simulink model "PassengerCar"  (R2019b)
settings: Solver=ode1  StartTime=0  StopTime=25  FixedStep=1.0000000000000000e-003  RelTol=1e-3
InitFcn:
  | sampleTime = str2double(get_param(bdroot, 'FixedStep'));
undefined symbols (not defined in the file or in its folder): AccPedalPos, BrakePedalPos, BrakeSwitch, DiscIntNeverNeededParam, DYNA4, EngSpd, IgnitionSwitch, InitialGear, InitialSpeed, IntendedEngTrq, LeftIndicator, MainBrakePress, MaxGear, MDL, MinGear, RefAcc, RefLane, RefLatPos, RefPath, RefPathCurv, RefSpd, RefSpdPreview, RefSpdRetrospect, RightIndicator, SteeringWheelAng, SteeringWheelTrq, UserDefinedRefValue, vm_const
libraries: UtilitiesLibrary x31, simulink x18, WheelSystemModules x13, LongitudinalControllerModules x13, LateralControllerModules x7, AnimationBusselectorModules x5, EnvironmentModules x5, BasicEngineControlModules x5, MiscellaneousControlModules x5, Animation3Modules x4, AuxiliariesModules x4, TireModules x4
(part 17 of 39)

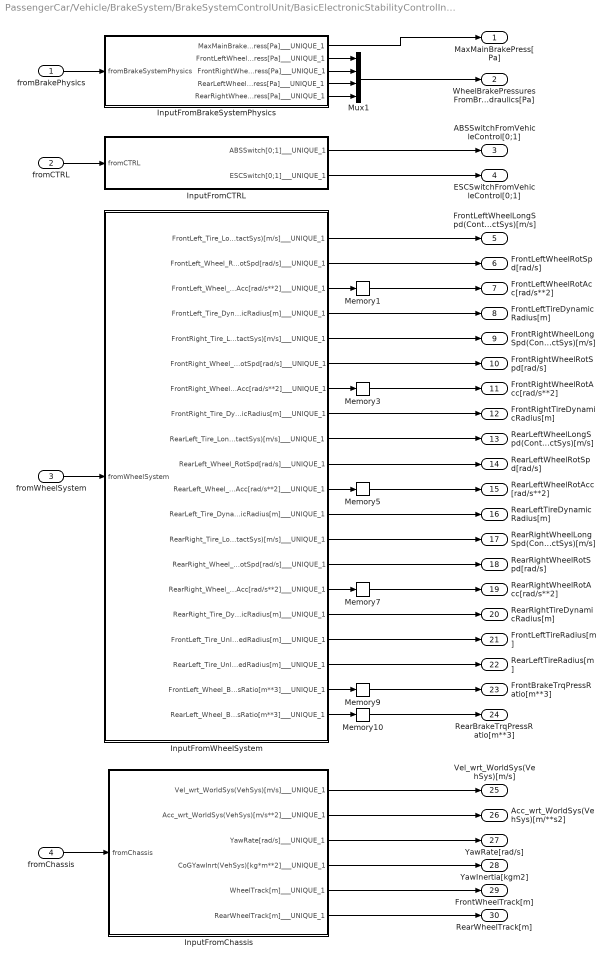
== system PassengerCar/Vehicle/BrakeSystem/BrakeSystemControlUnit/BasicElectronicStabilityControlInput ==
  fromBrakePhysics : Inport
  fromCTRL : Inport  Port=2
  fromWheelSystem : Inport  Port=3
  fromChassis : Inport  Port=4
  InputFromBrakeSystemPhysics : Subsystem  Tag=TESIS DYNAware Interface Block  mask{NeedsUpdate=off, SignalInfo=|}
      mask SignalInfo=|
      | {
      |   "Version": "4.6",
      |   "MuxedOutputBusName": "output",
      |   "MuxedInputBusName": "fromBrakeSystemPhysics",
      |   "MuxedInputSelected": true,
      |   "MuxedOutputSelected": false,
      |   "SignalData": [
      |     {
      |       "initialValue": "",
      |       "name": "MaxMainBrakePress[Pa]",
      |       "comment": "",
      |       "minString": "",
      |       "maxString": "",
      |       "width": -1,
      |       "dataType": 0,
      |       "signalType": 0,
      |       "createSignal": false,
      |       "outputName": "MaxMainBrakePress[Pa]",
      |       "generateSignalAccessBlock": false,
      |       "accessId": "$(parentId).$(blockName).$(outputName)"
      |     },
      |     {
      |       "initialValue": "",
      |       "name": "FrontLeftWheelBrakePress[Pa]",
      |       "comment": "",
      |       "minString": "",
      |       "maxString": "",
      |       "width": -1,
      |       "dataType": 0,
      |       "signalType": 0,
      |       "createSignal": false,
      |       "outputName": "FrontLeftWheelBrakePress[Pa]",
      |       "generateSignalAccessBlock": false,
      |       "accessId": "$(parentId).$(blockName).$(outputName)"
      |     },
      |     {
      |       "initialValue": "",
      |       "name": "FrontRightWheelBrakePress[Pa]",
      |       "comment": "",
      |       "minString": "",
      |       "maxString": "",
      |       "width": -1,
      |       "dataType": 0,
      |       "signalType": 0,
      |       "createSignal": false,
      |       "outputName": "FrontRightWheelBrakePress[Pa]",
      |       "generateSignalAccessBlock": false,
      |       "accessId": "$(parentId).$(blockName).$(outputName)"
      |     },
      |     {
      |       "initialValue": "",
      |       "name": "RearLeftWheelBrakePress[Pa]",
      |       "comment": "",
      |       "minString": "",
      |       "maxString": "",
      |       "width": -1,
      |       "dataType": 0,
      |       "signalType": 0,
      |       "createSignal": false,
      |       "outputName": "RearLeftWheelBrakePress[Pa]",
      |       "generateSignalAccessBlock": false,
      |       "accessId": "$(parentId).$(blockName).$(outputName)"
      |     },
      |     {
      |       "initialValue": "",
      |       "name": "RearRightWheelBrakePress[Pa]",
      |       "comment": "",
      |       "minString": "",
      |       "maxString": "",
      |       "width": -1,
      |       "dataType": 0,
      |       "signalType": 0,
      |       "createSignal": false,
      |       "outputName": "RearRightWheelBrakePress[Pa]",
      |       "generateSignalAccessBlock": false,
      |       "accessId": "$(parentId).$(blockName).$(outputName)"
      |     }
      |   ]
      | }
      mask prompts: NeedsUpdate "Specify, if subsystem content needs to be updated"; SignalInfo "Signal Info (json)"
      mask help: DYNA4 Interface Block Version 4.6
      mask init:
      | blockName = get_param(gcbh, 'Name');
      | parentId = DYNA4.ModelHandling.AccessID.getFromHierarchy(gcbh);
      | TD.InterfaceBlock.ModelCallbacks.GenerateContent(gcb);
      settings: DeleteFcn=TD.InterfaceBlock.ModelCallbacks.CloseGUI( gcbh );  NameChangeFcn=TD.InterfaceBlock.ModelCallbacks.BlockRenamedHandler(gcbh);  OpenFcn=TD.InterfaceBlock.ModelCallbacks.OpenGUI( gcbh );  CloseFcn=TD.InterfaceBlock.ModelCallbacks.CloseGUI( gcbh );
      mask Display:
      | image('InterfaceBlock.png','center');
      | port_label('input',1, 'fromBrakeSystemPhysics');
      | port_label('output',1, 'MaxMainBrakePress[Pa]');
      | port_label('output',2, 'FrontLeftWheelBrakePress[Pa]');
      | port_label('output',3, 'FrontRightWheelBrakePress[Pa]');
      | port_label('output',4, 'RearLeftWheelBrakePress[Pa]');
      | port_label('output',5, 'RearRightWheelBrakePress[Pa]');
  InputFromCTRL : Subsystem  Tag=TESIS DYNAware Interface Block  mask{NeedsUpdate=off, SignalInfo=|}
      mask SignalInfo=|
      | {
      |   "Version": "4.6",
      |   "MuxedOutputBusName": "output",
      |   "MuxedInputBusName": "fromCTRL",
      |   "MuxedInputSelected": true,
      |   "MuxedOutputSelected": false,
      |   "SignalData": [
      |     {
      |       "initialValue": "0.0",
      |       "name": "CTRL.LongitudinalControl.ABSSwitch[0;1]",
      |       "comment": "",
      |       "minString": "",
      |       "maxString": "",
      |       "width": 1,
      |       "dataType": 0,
      |       "signalType": 0,
      |       "createSignal": false,
      |       "outputName": "ABSSwitch[0;1]",
      |       "generateSignalAccessBlock": false,
      |       "accessId": "$(parentId).$(blockName).$(outputName)"
      |     },
      |     {
      |       "initialValue": "0.0",
      |       "name": "CTRL.LongitudinalControl.ESCSwitch[0;1]",
      |       "comment": "",
      |       "minString": "",
      |       "maxString": "",
      |       "width": 1,
      |       "dataType": 0,
      |       "signalType": 0,
      |       "createSignal": false,
      |       "outputName": "ESCSwitch[0;1]",
      |       "generateSignalAccessBlock": false,
      |       "accessId": "$(parentId).$(blockName).$(outputName)"
      |     }
      |   ]
      | }
      mask prompts: NeedsUpdate "Specify, if subsystem content needs to be updated"; SignalInfo "Signal Info (json)"
      mask help: DYNA4 Interface Block Version 4.6
      mask init:
      | blockName = get_param(gcbh, 'Name');
      | parentId = DYNA4.ModelHandling.AccessID.getFromHierarchy(gcbh);
      | TD.InterfaceBlock.ModelCallbacks.GenerateContent(gcb);
      settings: DeleteFcn=TD.InterfaceBlock.ModelCallbacks.CloseGUI( gcbh );  NameChangeFcn=TD.InterfaceBlock.ModelCallbacks.BlockRenamedHandler(gcbh);  OpenFcn=TD.InterfaceBlock.ModelCallbacks.OpenGUI( gcbh );  CloseFcn=TD.InterfaceBlock.ModelCallbacks.CloseGUI( gcbh );
      mask Display:
      | image('InterfaceBlock.png','center');
      | port_label('input',1, 'fromCTRL');
      | port_label('output',1, 'ABSSwitch[0;1]');
      | port_label('output',2, 'ESCSwitch[0;1]');
  InputFromChassis : Subsystem  Tag=TESIS DYNAware Interface Block  mask{NeedsUpdate=off, SignalInfo=|}
      mask SignalInfo=|
      | {
      |   "Version": "4.6",
      |   "MuxedOutputBusName": "output",
      |   "MuxedInputBusName": "fromChassis",
      |   "MuxedInputSelected": true,
      |   "MuxedOutputSelected": false,
      |   "SignalData": [
      |     {
      |       "initialValue": "0.0",
      |       "name": "VehicleBody.Vel_wrt_WorldSys(VehSys)[m/s]",
      |       "comment": "",
      |       "minString": "",
      |       "maxString": "",
      |       "width": 3,
      |       "dataType": 0,
      |       "signalType": 0,
      |       "createSignal": false,
      |       "outputName": "Vel_wrt_WorldSys(VehSys)[m/s]",
      |       "generateSignalAccessBlock": false,
      |       "accessId": "$(parentId).$(blockName).$(outputName)"
      |     },
      |     {
      |       "initialValue": "0.0",
      |       "name": "VehicleBody.Acc_wrt_WorldSys(VehSys)[m/s**2]",
      |       "comment": "",
      |       "minString": "",
      |       "maxString": "",
      |       "width": 3,
      |       "dataType": 0,
      |       "signalType": 0,
      |       "createSignal": false,
      |       "outputName": "Acc_wrt_WorldSys(VehSys)[m/s**2]",
      |       "generateSignalAccessBlock": false,
      |       "accessId": "$(parentId).$(blockName).$(outputName)"
      |     },
      |     {
      |       "initialValue": "0.0",
      |       "name": "VehicleBody.YawRate[rad/s]",
      |       "comment": "",
      |       "minString": "",
      |       "maxString": "",
      |       "width": 1,
      |       "dataType": 0,
      |       "signalType": 0,
      |       "createSignal": false,
      |       "outputName": "YawRate[rad/s]",
      |       "generateSignalAccessBlock": false,
      |       "accessId": "$(parentId).$(blockName).$(outputName)"
      |     },
      |     {
      |       "initialValue": "0.0",
      |       "name": "VehicleBody.CoGYawInrt(VehSys)[kg*m**2]",
      |       "comment": "",
      |       "minString": "",
      |       "maxString": "",
      |       "width": 1,
      |       "dataType": 0,
      |       "signalType": 0,
      |       "createSignal": false,
      |       "outputName": "CoGYawInrt(VehSys)[kg*m**2]",
      |       "generateSignalAccessBlock": false,
      |       "accessId": "$(parentId).$(blockName).$(outputName)"
      |     },
      |     {
      |       "initialValue": "0.0",
      |       "name": "FrontAxle.WheelTrack[m]",
      |       "comment": "",
      |       "minString": "",
      |       "maxString": "",
      |       "width": 1,
      |       "dataType": 0,
      |       "signalType": 0,
      |       "createSignal": false,
      |       "outputName": "WheelTrack[m]",
      |       "generateSignalAccessBlock": false,
      |       "accessId": "$(parentId).$(blockName).$(outputName)"
      |     },
      |     {
      |       "initialValue": "0.0",
      |       "name": "RearAxle.WheelTrack[m]",
      |       "comment": "",
      |       "minString": "",
      |       "maxString": "",
      |       "width": 1,
      |       "dataType": 0,
      |       "signalType": 0,
      |       "createSignal": false,
      |       "outputName": "RearWheelTrack[m]",
      |       "generateSignalAccessBlock": false,
      |       "accessId": "$(parentId).$(blockName).$(outputName)"
      |     }
      |   ]
      | }
      mask prompts: NeedsUpdate "Specify, if subsystem content needs to be updated"; SignalInfo "Signal Info (json)"
      mask help: DYNA4 Interface Block Version 4.6
      mask init:
      | blockName = get_param(gcbh, 'Name');
      | parentId = DYNA4.ModelHandling.AccessID.getFromHierarchy(gcbh);
      | TD.InterfaceBlock.ModelCallbacks.GenerateContent(gcb);
      settings: DeleteFcn=TD.InterfaceBlock.ModelCallbacks.CloseGUI( gcbh );  NameChangeFcn=TD.InterfaceBlock.ModelCallbacks.BlockRenamedHandler(gcbh);  OpenFcn=TD.InterfaceBlock.ModelCallbacks.OpenGUI( gcbh );  CloseFcn=TD.InterfaceBlock.ModelCallbacks.CloseGUI( gcbh );
      mask Display:
      | image('InterfaceBlock.png','center');
      | port_label('input',1, 'fromChassis');
      | port_label('output',1, 'Vel_wrt_WorldSys(VehSys)[m/s]');
      | port_label('output',2, 'Acc_wrt_WorldSys(VehSys)[m/s**2]');
      | port_label('output',3, 'YawRate[rad/s]');
      | port_label('output',4, 'CoGYawInrt(VehSys)[kg*m**2]');
      | port_label('output',5, 'WheelTrack[m]');
      | port_label('output',6, 'RearWheelTrack[m]');
  InputFromWheelSystem : Subsystem  Tag=TESIS DYNAware Interface Block  mask{NeedsUpdate=off, SignalInfo=|}
      mask SignalInfo=|
      | {
      |   "Version": "4.6",
      |   "MuxedOutputBusName": "output",
      |   "MuxedInputBusName": "fromWheelSystem",
      |   "MuxedInputSelected": true,
      |   "MuxedOutputSelected": false,
      |   "SignalData": [
      |     {
      |       "initialValue": "0.0",
      |       "name": "FrontLeft.Tire.LongSpd(ContactSys)[m/s]",
      |       "comment": "Front left longitudinal wheel speed in contact system",
      |       "minString": "",
      |       "maxString": "",
      |       "width": 1,
      |       "dataType": 0,
      |       "signalType": 0,
      |       "createSignal": false,
      |       "outputName": "FrontLeft_Tire_LongSpd(ContactSys)[m/s]",
      |       "generateSignalAccessBlock": false,
      |       "accessId": "$(parentId).$(blockName).$(outputName)"
      |     },
      |     {
      |       "initialValue": "0.0",
      |       "name": "FrontLeft.Wheel.RotSpd[rad/s]",
      |       "comment": "Front left wheel rotational speed",
      |       "minString": "",
      |       "maxString": "",
      |       "width": -1,
      |       "dataType": 0,
      |       "signalType": 0,
      |       "createSignal": false,
      |       "outputName": "FrontLeft_Wheel_RotSpd[rad/s]",
      |       "generateSignalAccessBlock": false,
      |       "accessId": "$(parentId).$(blockName).$(outputName)"
      |     },
      |     {
      |       "initialValue": "0.0",
      |       "name": "FrontLeft.Wheel.RotAcc[rad/s**2]",
      |       "comment": "Front left wheel rotational acceleration",
      |       "minString": "",
      |       "maxString": "",
      |       "width": 1,
      |       "dataType": 0,
      |       "signalType": 0,
      |       "createSignal": false,
      |       "outputName": "FrontLeft_Wheel_RotAcc[rad/s**2]",
      |       "generateSignalAccessBlock": false,
      |       "accessId": "$(parentId).$(blockName).$(outputName)"
      |     },
      |     {
      |       "initialValue": "0.0",
      |       "name": "FrontLeft.Tire.DynamicRadius[m]",
      |       "comment": "Front left tire dynamic radius",
      |       "minString": "",
      |       "maxString": "",
      |       "width": 1,
      |       "dataType": 0,
      |       "signalType": 0,
      |       "createSignal": false,
      |       "outputName": "FrontLeft_Tire_DynamicRadius[m]",
      |       "generateSignalAccessBlock": false,
      |       "accessId": "$(parentId).$(blockName).$(outputName)"
      |     },
      |     {
      |       "initialValue": "0.0",
      |       "name": "FrontRight.Tire.LongSpd(ContactSys)[m/s]",
      |       "comment": "Front right wheel longitudinal speed in contact system",
      |       "minString": "",
      |       "maxString": "",
      |       "width": 1,
      |       "dataType": 0,
      |       "signalType": 0,
      |       "createSignal": false,
      |       "outputName": "FrontRight_Tire_LongSpd(ContactSys)[m/s]",
      |       "generateSignalAccessBlock": false,
      |       "accessId": "$(parentId).$(blockName).$(outputName)"
      |     },
      |     {
      |       "initialValue": "0.0",
      |       "name": "FrontRight.Wheel.RotSpd[rad/s]",
      |       "comment": "Front right wheel rotational speed",
      |       "minString": "",
      |       "maxString": "",
      |       "width": 1,
      |       "dataType": 0,
      |       "signalType": 0,
      |       "createSignal": false,
      |       "outputName": "FrontRight_Wheel_RotSpd[rad/s]",
      |       "generateSignalAccessBlock": false,
      |       "accessId": "$(parentId).$(blockName).$(outputName)"
      |     },
      |     {
      |       "initialValue": "0.0",
      |       "name": "FrontRight.Wheel.RotAcc[rad/s**2]",
      |       "comment": "Front right wheel rotational acceleration",
      |       "minString": "",
      |       "maxString": "",
      |       "width": 1,
      |       "dataType": 0,
      |       "signalType": 0,
      |       "createSignal": false,
      |       "outputName": "FrontRight_Wheel_RotAcc[rad/s**2]",
      |       "generateSignalAccessBlock": false,
      |       "accessId": "$(parentId).$(blockName).$(outputName)"
      |     },
      |     {
      |       "initialValue": "0.0",
      |       "name": "FrontRight.Tire.DynamicRadius[m]",
      |       "comment": "Front right tire dynamic radius",
      |       "minString": "",
      |       "maxString": "",
      |       "width": 1,
      |       "dataType": 0,
      |       "signalType": 0,
      |       "createSignal": false,
      |       "outputName": "FrontRight_Tire_DynamicRadius[m]",
      |       "generateSignalAccessBlock": false,
      |       "accessId": "$(parentId).$(blockName).$(outputName)"
      |     },
      |     {
      |       "initialValue": "0.0",
      |       "name": "RearLeft.Tire.LongSpd(ContactSys)[m/s]",
      |       "comment": "Rear left wheel longitudinal speed in contact system",
      |       "minString": "",
      |       "maxString": "",
      |       "width": 1,
      |       "dataType": 0,
      |       "signalType": 0,
      |       "createSignal": false,
      |       "outputName": "RearLeft_Tire_LongSpd(ContactSys)[m/s]",
      |       "generateSignalAccessBlock": false,
      |       "accessId": "$(parentId).$(blockName).$(outputName)"
      |     },
      |     {
      |       "initialValue": "0.0",
      |       "name": "RearLeft.Wheel.RotSpd[rad/s]",
      |       "comment": "Rear left wheel rotational speed",
      |       "minString": "",
      |       "maxString": "",
      |       "width": 1,
      |       "dataType": 0,
      |       "signalType": 0,
      |       "createSignal": false,
      |       "outputName": "RearLeft_Wheel_RotSpd[rad/s]",
      |       "generateSignalAccessBlock": false,
      |       "accessId": "$(parentId).$(blockName).$(outputName)"
      |     },
      |     {
      |       "initialValue": "0.0",
      |       "name": "RearLeft.Wheel.RotAcc[rad/s**2]",
      |       "comment": "Rear left wheel rotational acceleration",
      |       "minString": "",
      |       "maxString": "",
      |       "width": 1,
      |       "dataType": 0,
      |       "signalType": 0,
      |       "createSignal": false,
      |       "outputName": "RearLeft_Wheel_RotAcc[rad/s**2]",
      |       "generateSignalAccessBlock": false,
      |       "accessId": "$(parentId).$(blockName).$(outputName)"
      |     },
      |     {
      |       "initialValue": "0.0",
      |       "name": "RearLeft.Tire.DynamicRadius[m]",
      |       "comment": "Rear left tire dynamic radius",
      |       "minString": "",
      |       "maxString": "",
      |       "width": 1,
      |       "dataType": 0,
      |       "signalType": 0,
      |       "createSignal": false,
      |       "outputName": "RearLeft_Tire_DynamicRadius[m]",
      |       "generateSignalAccessBlock": false,
      |       "accessId": "$(parentId).$(blockName).$(outputName)"
      |     },
      |     {
      |       "initialValue": "0.0",
      |       "name": "RearRight.Tire.LongSpd(ContactSys)[m/s]",
      |       "comment": "Rear right wheel longitudinal speed in contact system",
      |       "minString": "",
      |       "maxString": "",
      |       "width": 1,
      |       "dataType": 0,
      |       "signalType": 0,
      |       "createSignal": false,
      |       "outputName": "RearRight_Tire_LongSpd(ContactSys)[m/s]",
      |       "generateSignalAccessBlock": false,
      |       "accessId": "$(parentId).$(blockName).$(outputName)"
      |     },
      |     {
      |       "initialValue": "0.0",
      |       "name": "RearRight.Wheel.RotSpd[rad/s]",
      |       "comment": "Rear right wheel rotational speed",
      |       "minString": "",
      |       "maxString": "",
      |       "width": 1,
      |       "dataType": 0,
      |       "signalType": 0,
      |       "createSignal": false,
      |       "outputName": "RearRight_Wheel_RotSpd[rad/s]",
      |       "generateSignalAccessBlock": false,
      |       "accessId": "$(parentId).$(blockName).$(outputName)"
      |     },
      |     {
      |       "initialValue": "0.0",
      |       "name": "RearRight.Wheel.RotAcc[rad/s**2]",
      |       "comment": "Rear right wheel rotational acceleration",
      |       "minString": "",
      |       "maxString": "",
      |       "width": 1,
      |       "dataType": 0,
      |       "signalType": 0,
      |       "createSignal": false,
      |       "outputName": "RearRight_Wheel_RotAcc[rad/s**2]",
      |       "generateSignalAccessBlock": false,
      |       "accessId": "$(parentId).$(blockName).$(outputName)"
      |     },
      |     {
      |       "initialValue": "0.0",
      |       "name": "RearRight.Tire.DynamicRadius[m]",
      |       "comment": "Rear right tire dynamic radius",
      |       "minString": "",
      |       "maxString": "",
      |       "width": 1,
      |       "dataType": 0,
      |       "signalType": 0,
      |       "createSignal": false,
      |       "outputName": "RearRight_Tire_DynamicRadius[m]",
      |       "generateSignalAccessBlock": false,
      |       "accessId": "$(parentId).$(blockName).$(outputName)"
      |     },
      |     {
      |       "initialValue": "0.0",
      |       "name": "FrontLeft.Tire.UnloadedRadius[m]",
      |       "comment": "",
      |       "minString": "",
      |       "maxString": "",
      |       "width": 1,
      |       "dataType": 0,
      |       "signalType": 0,
      |       "createSignal": false,
      |       "outputName": "FrontLeft_Tire_UnloadedRadius[m]",
      |       "generateSignalAccessBlock": false,
      |       "accessId": "$(parentId).$(blockName).$(outputName)"
      |     },
      |     {
      |       "initialValue": "0.0",
      |       "name": "RearLeft.Tire.UnloadedRadius[m]",
      |       "comment": "",
      |       "minString": "",
      |       "maxString": "",
      |       "width": 1,
      |       "dataType": 0,
      |       "signalType": 0,
      |       "createSignal": false,
      |       "outputName": "RearLeft_Tire_UnloadedRadius[m]",
      |       "generateSignalAccessBlock": false,
      |       "accessId": "$(parentId).$(blockName).$(outputName)"
      |     },
      |     {
      |       "initialValue": "0.0",
      |       "name": "FrontLeft.Wheel.BrakeTrqPressRatio[m**3]",
      |       "comment": "",
      |       "minString": "",
      |       "maxString": "",
      |       "width": 1,
      |       "dataType": 0,
      |       "signalType": 0,
      |       "createSignal": false,
      |       "outputName": "FrontLeft_Wheel_BrakeTrqPressRatio[m**3]",
      |       "generateSignalAccessBlock": false,
      |       "accessId": "$(parentId).$(blockName).$(outputName)"
      |     },
      |     {
      |       "initialValue": "0.0",
      |       "name": "RearLeft.Wheel.BrakeTrqPressRatio[m**3]",
      |       "comment": "",
      |       "minString": "",
      |       "maxString": "",
      |       "width": 1,
      |       "dataType": 0,
      |       "signalType": 0,
      |       "createSignal": false,
      |       "outputName": "RearLeft_Wheel_BrakeTrqPressRatio[m**3]",
      |       "generateSignalAccessBlock": false,
      |       "accessId": "$(parentId).$(blockName).$(outputName)"
      |     }
      |   ]
      | }
      mask prompts: NeedsUpdate "Specify, if subsystem content needs to be updated"; SignalInfo "Signal Info (json)"
      mask help: DYNA4 Interface Block Version 4.6
      mask init:
      | blockName = get_param(gcbh, 'Name');
      | parentId = DYNA4.ModelHandling.AccessID.getFromHierarchy(gcbh);
      | TD.InterfaceBlock.ModelCallbacks.GenerateContent(gcb);
      settings: DeleteFcn=TD.InterfaceBlock.ModelCallbacks.CloseGUI( gcbh );  NameChangeFcn=TD.InterfaceBlock.ModelCallbacks.BlockRenamedHandler(gcbh);  OpenFcn=TD.InterfaceBlock.ModelCallbacks.OpenGUI( gcbh );  CloseFcn=TD.InterfaceBlock.ModelCallbacks.CloseGUI( gcbh );
      mask Display:
      | image('InterfaceBlock.png','center');
      | port_label('input',1, 'fromWheelSystem');
      | port_label('output',1, 'FrontLeft_Tire_LongSpd(ContactSys)[m/s]');
      | port_label('output',2, 'FrontLeft_Wheel_RotSpd[rad/s]');
      | port_label('output',3, 'FrontLeft_Wheel_RotAcc[rad/s**2]');
      | port_label('output',4, 'FrontLeft_Tire_DynamicRadius[m]');
      | port_label('output',5, 'FrontRight_Tire_LongSpd(ContactSys)[m/s]');
      | port_label('output',6, 'FrontRight_Wheel_RotSpd[rad/s]');
      | port_label('output',7, 'FrontRight_Wheel_RotAcc[rad/s**2]');
      | port_label('output',8, 'FrontRight_Tire_DynamicRadius[m]');
      | port_label('output',9, 'RearLeft_Tire_LongSpd(ContactSys)[m/s]');
      | port_label('output',10, 'RearLeft_Wheel_RotSpd[rad/s]');
      | port_label('output',11, 'RearLeft_Wheel_RotAcc[rad/s**2]');
      | port_label('output',12, 'RearLeft_Tire_DynamicRadius[m]');
      | port_label('output',13, 'RearRight_Tire_LongSpd(ContactSys)[m/s]');
      | port_label('output',14, 'RearRight_Wheel_RotSpd[rad/s]');
      | port_label('output',15, 'RearRight_Wheel_RotAcc[rad/s**2]');
      | port_label('output',16, 'RearRight_Tire_DynamicRadius[m]');
      | port_label('output',17, 'FrontLeft_Tire_UnloadedRadius[m]');
      | port_label('output',18, 'RearLeft_Tire_UnloadedRadius[m]');
      | port_label('output',19, 'FrontLeft_Wheel_BrakeTrqPressRatio[m**3]');
      | port_label('output',20, 'RearLeft_Wheel_BrakeTrqPressRatio[m**3]');
  Memory{1,3,5,7,9..10} (6 alike) : Memory  InheritSampleTime=on
  Mux1 : Mux
  MaxMainBrakePress[Pa] : Outport  VectorParamsAs1DForOutWhenUnconnected=off
  WheelBrakePressuresFromBrakeHydraulics[Pa] : Outport  Port=2  VectorParamsAs1DForOutWhenUnconnected=off
  ABSSwitchFromVehicleControl[0;1] : Outport  Port=3  VectorParamsAs1DForOutWhenUnconnected=off
  ESCSwitchFromVehicleControl[0;1] : Outport  Port=4  VectorParamsAs1DForOutWhenUnconnected=off
  FrontLeftWheelLongSpd(ContactSys)[m/s] : Outport  Port=5  VectorParamsAs1DForOutWhenUnconnected=off
  FrontLeftWheelRotSpd[rad/s] : Outport  Port=6  VectorParamsAs1DForOutWhenUnconnected=off
  FrontLeftWheelRotAcc[rad/s**2] : Outport  Port=7  VectorParamsAs1DForOutWhenUnconnected=off
  FrontLeftTireDynamicRadius[m] : Outport  Port=8  VectorParamsAs1DForOutWhenUnconnected=off
  FrontRightWheelLongSpd(ContactSys)[m/s] : Outport  Port=9  VectorParamsAs1DForOutWhenUnconnected=off
  FrontRightWheelRotSpd[rad/s] : Outport  Port=10  VectorParamsAs1DForOutWhenUnconnected=off
  FrontRightWheelRotAcc[rad/s**2] : Outport  Port=11  VectorParamsAs1DForOutWhenUnconnected=off
  FrontRightTireDynamicRadius[m] : Outport  Port=12  VectorParamsAs1DForOutWhenUnconnected=off
  RearLeftWheelLongSpd(ContactSys)[m/s] : Outport  Port=13  VectorParamsAs1DForOutWhenUnconnected=off
  RearLeftWheelRotSpd[rad/s] : Outport  Port=14  VectorParamsAs1DForOutWhenUnconnected=off
  RearLeftWheelRotAcc[rad/s**2] : Outport  Port=15  VectorParamsAs1DForOutWhenUnconnected=off
  RearLeftTireDynamicRadius[m] : Outport  Port=16  VectorParamsAs1DForOutWhenUnconnected=off
  RearRightWheelLongSpd(ContactSys)[m/s] : Outport  Port=17  VectorParamsAs1DForOutWhenUnconnected=off
  RearRightWheelRotSpd[rad/s] : Outport  Port=18  VectorParamsAs1DForOutWhenUnconnected=off
  RearRightWheelRotAcc[rad/s**2] : Outport  Port=19  VectorParamsAs1DForOutWhenUnconnected=off
  RearRightTireDynamicRadius[m] : Outport  Port=20  VectorParamsAs1DForOutWhenUnconnected=off
  FrontLeftTireRadius[m] : Outport  Port=21  VectorParamsAs1DForOutWhenUnconnected=off
  RearLeftTireRadius[m] : Outport  Port=22  VectorParamsAs1DForOutWhenUnconnected=off
  FrontBrakeTrqPressRatio[m**3] : Outport  Port=23  VectorParamsAs1DForOutWhenUnconnected=off
  RearBrakeTrqPressRatio[m**3] : Outport  Port=24  VectorParamsAs1DForOutWhenUnconnected=off
  Vel_wrt_WorldSys(VehSys)[m/s] : Outport  Port=25  VectorParamsAs1DForOutWhenUnconnected=off
  Acc_wrt_WorldSys(VehSys)[m/**s2] : Outport  Port=26  VectorParamsAs1DForOutWhenUnconnected=off
  YawRate[rad/s] : Outport  Port=27  VectorParamsAs1DForOutWhenUnconnected=off
  YawInertia[kgm2] : Outport  Port=28  VectorParamsAs1DForOutWhenUnconnected=off
  FrontWheelTrack[m] : Outport  Port=29  VectorParamsAs1DForOutWhenUnconnected=off
  RearWheelTrack[m] : Outport  Port=30  VectorParamsAs1DForOutWhenUnconnected=off
  wires:
  Memory3/1 -> FrontRightWheelRotAcc[rad/s**2]/1
  InputFromWheelSystem/9(RearLeft_Tire_LongSpd(ContactSys)[m/s]___UNIQUE_1) -> RearLeftWheelLongSpd(ContactSys)[m/s]/1
  InputFromWheelSystem/6(FrontRight_Wheel_RotSpd[rad/s]___UNIQUE_1) -> FrontRightWheelRotSpd[rad/s]/1
  InputFromChassis/5(WheelTrack[m]___UNIQUE_1) -> FrontWheelTrack[m]/1
  InputFromWheelSystem/20(RearLeft_Wheel_BrakeTrqPressRatio[m**3]___UNIQUE_1) -> Memory10/1
  InputFromChassis/4(CoGYawInrt(VehSys)[kg*m**2]___UNIQUE_1) -> YawInertia[kgm2]/1
  fromCTRL/1 -> InputFromCTRL/1(fromCTRL)
  InputFromWheelSystem/16(RearRight_Tire_DynamicRadius[m]___UNIQUE_1) -> RearRightTireDynamicRadius[m]/1
  InputFromWheelSystem/1(FrontLeft_Tire_LongSpd(ContactSys)[m/s]___UNIQUE_1) -> FrontLeftWheelLongSpd(ContactSys)[m/s]/1
  InputFromCTRL/2(ESCSwitch[0;1]___UNIQUE_1) -> ESCSwitchFromVehicleControl[0;1]/1
  InputFromWheelSystem/14(RearRight_Wheel_RotSpd[rad/s]___UNIQUE_1) -> RearRightWheelRotSpd[rad/s]/1
  fromWheelSystem/1 -> InputFromWheelSystem/1(fromWheelSystem)
  Memory1/1 -> FrontLeftWheelRotAcc[rad/s**2]/1
  InputFromWheelSystem/2(FrontLeft_Wheel_RotSpd[rad/s]___UNIQUE_1) -> FrontLeftWheelRotSpd[rad/s]/1
  fromChassis/1 -> InputFromChassis/1(fromChassis)
  InputFromWheelSystem/10(RearLeft_Wheel_RotSpd[rad/s]___UNIQUE_1) -> RearLeftWheelRotSpd[rad/s]/1
  InputFromWheelSystem/11(RearLeft_Wheel_RotAcc[rad/s**2]___UNIQUE_1) -> Memory5/1
  InputFromWheelSystem/19(FrontLeft_Wheel_BrakeTrqPressRatio[m**3]___UNIQUE_1) -> Memory9/1
  InputFromWheelSystem/17(FrontLeft_Tire_UnloadedRadius[m]___UNIQUE_1) -> FrontLeftTireRadius[m]/1
  InputFromWheelSystem/12(RearLeft_Tire_DynamicRadius[m]___UNIQUE_1) -> RearLeftTireDynamicRadius[m]/1
  InputFromWheelSystem/15(RearRight_Wheel_RotAcc[rad/s**2]___UNIQUE_1) -> Memory7/1
  InputFromChassis/3(YawRate[rad/s]___UNIQUE_1) -> YawRate[rad/s]/1
  InputFromWheelSystem/13(RearRight_Tire_LongSpd(ContactSys)[m/s]___UNIQUE_1) -> RearRightWheelLongSpd(ContactSys)[m/s]/1
  InputFromWheelSystem/3(FrontLeft_Wheel_RotAcc[rad/s**2]___UNIQUE_1) -> Memory1/1
  InputFromWheelSystem/18(RearLeft_Tire_UnloadedRadius[m]___UNIQUE_1) -> RearLeftTireRadius[m]/1
  InputFromCTRL/1(ABSSwitch[0;1]___UNIQUE_1) -> ABSSwitchFromVehicleControl[0;1]/1
  InputFromChassis/2(Acc_wrt_WorldSys(VehSys)[m/s**2]___UNIQUE_1) -> Acc_wrt_WorldSys(VehSys)[m/**s2]/1
  InputFromWheelSystem/4(FrontLeft_Tire_DynamicRadius[m]___UNIQUE_1) -> FrontLeftTireDynamicRadius[m]/1
  InputFromWheelSystem/5(FrontRight_Tire_LongSpd(ContactSys)[m/s]___UNIQUE_1) -> FrontRightWheelLongSpd(ContactSys)[m/s]/1
  Memory9/1 -> FrontBrakeTrqPressRatio[m**3]/1
  InputFromChassis/1(Vel_wrt_WorldSys(VehSys)[m/s]___UNIQUE_1) -> Vel_wrt_WorldSys(VehSys)[m/s]/1
  InputFromWheelSystem/7(FrontRight_Wheel_RotAcc[rad/s**2]___UNIQUE_1) -> Memory3/1
  Memory7/1 -> RearRightWheelRotAcc[rad/s**2]/1
  Memory10/1 -> RearBrakeTrqPressRatio[m**3]/1
  InputFromWheelSystem/8(FrontRight_Tire_DynamicRadius[m]___UNIQUE_1) -> FrontRightTireDynamicRadius[m]/1
  Memory5/1 -> RearLeftWheelRotAcc[rad/s**2]/1
  InputFromChassis/6(RearWheelTrack[m]___UNIQUE_1) -> RearWheelTrack[m]/1
  InputFromBrakeSystemPhysics/1(MaxMainBrakePress[Pa]___UNIQUE_1) -> MaxMainBrakePress[Pa]/1
  Mux1/1 -> WheelBrakePressuresFromBrakeHydraulics[Pa]/1
  InputFromBrakeSystemPhysics/3(FrontRightWheelBrakePress[Pa]___UNIQUE_1) -> Mux1/2
  InputFromBrakeSystemPhysics/2(FrontLeftWheelBrakePress[Pa]___UNIQUE_1) -> Mux1/1
  fromBrakePhysics/1 -> InputFromBrakeSystemPhysics/1(fromBrakeSystemPhysics)
  InputFromBrakeSystemPhysics/4(RearLeftWheelBrakePress[Pa]___UNIQUE_1) -> Mux1/3
  InputFromBrakeSystemPhysics/5(RearRightWheelBrakePress[Pa]___UNIQUE_1) -> Mux1/4

== system PassengerCar/Vehicle/BrakeSystem/BrakeSystemControlUnit/BrakeSystemControlUnitOutput ==
  FrontLeftWheelBrakePress[Pa]___UNIQUE_1 : Inport  Description=|  PortDimensions=[1]
      | <name>FrontLeftWheelBrakePress[Pa]</name>
      | <comment>Front left wheel brake pressure</comment>
  FrontRightWheelBrakePress[Pa]___UNIQUE_1 : Inport  Description=|  Port=2  PortDimensions=[1]
      | <name>FrontRightWheelBrakePress[Pa]</name>
      | <comment>Front right wheel brake pressure</comment>
  RearLeftWheelBrakePress[Pa]___UNIQUE_1 : Inport  Description=|  Port=3  PortDimensions=[1]
      | <name>RearLeftWheelBrakePress[Pa]</name>
      | <comment>Rear left wheel brake pressure</comment>
  RearRightWheelBrakePress[Pa]___UNIQUE_1 : Inport  Description=|  Port=4  PortDimensions=[1]
      | <name>RearRightWheelBrakePress[Pa]</name>
      | <comment>Rear right wheel brake pressure</comment>
  Rear2LeftWheelBrakePress[Pa]___UNIQUE_1 : Inport  Description=|  Port=5  PortDimensions=[1]
      | <name>Rear2LeftWheelBrakePress[Pa]</name>
      | <comment></comment>
  Rear2RightWheelBrakePress[Pa]___UNIQUE_1 : Inport  Description=|  Port=6  PortDimensions=[1]
      | <name>Rear2RightWheelBrakePress[Pa]</name>
      | <comment></comment>
  Rear3LeftWheelBrakePress[Pa]___UNIQUE_1 : Inport  Description=|  Port=7  PortDimensions=[1]
      | <name>Rear3LeftWheelBrakePress[Pa]</name>
      | <comment></comment>
  Rear3RightWheelBrakePress[Pa]___UNIQUE_1 : Inport  Description=|  Port=8  PortDimensions=[1]
      | <name>Rear3RightWheelBrakePress[Pa]</name>
      | <comment></comment>
  WheelBrakePressActive[0;1]___UNIQUE_1 : Inport  Description=|  Port=9  PortDimensions=[1]
      | <name>WheelBrakePressActive[0;1]</name>
      | <comment></comment>
  YawStabilityControl___UNIQUE_1 : Inport  Description=|  Port=10
      | <name>ControlUnit.YawStabilityControl</name>
      | <comment></comment>
  AntiLockBrakeSystem___UNIQUE_1 : Inport  Description=|  Port=11
      | <name>ControlUnit.AntiLockBrakeSystem</name>
      | <comment></comment>
  __TDD__BrakeSystemControlUnit.FrontLeftWheelBrakePress[Pa] : Demux  Outputs=[1]
  __TDD__BrakeSystemControlUnit.FrontRightWheelBrakePress[Pa] : Demux  Outputs=[1]
  __TDD__BrakeSystemControlUnit.Rear2LeftWheelBrakePress[Pa] : Demux  Outputs=[1]
  __TDD__BrakeSystemControlUnit.Rear2RightWheelBrakePress[Pa] : Demux  Outputs=[1]
  __TDD__BrakeSystemControlUnit.Rear3LeftWheelBrakePress[Pa] : Demux  Outputs=[1]
  __TDD__BrakeSystemControlUnit.Rear3RightWheelBrakePress[Pa] : Demux  Outputs=[1]
  __TDD__BrakeSystemControlUnit.RearLeftWheelBrakePress[Pa] : Demux  Outputs=[1]
  __TDD__BrakeSystemControlUnit.RearRightWheelBrakePress[Pa] : Demux  Outputs=[1]
  __TDD__BrakeSystemControlUnit.WheelBrakePressActive[0;1] : Demux  Outputs=[1]
  __TDO__BrakeSystemControlUnit : BusCreator  Inputs=10
  __TDO__BrakeSystemControlUnit.ControlUnit : BusCreator  Inputs=2
  BrakeSystemControlUnit___UNIQUE_1 : Outport  Description=|  VectorParamsAs1DForOutWhenUnconnected=off
      | <name>FrontLeftWheelBrakePress[Pa]</name>
      | <comment>Front left wheel brake pressure</comment>
  wires:
  FrontLeftWheelBrakePress[Pa]___UNIQUE_1/1 -> __TDD__BrakeSystemControlUnit.FrontLeftWheelBrakePress[Pa]/1  "FrontLeftWheelBrakePress[Pa]"
  __TDD__BrakeSystemControlUnit.FrontLeftWheelBrakePress[Pa]/1 -> __TDO__BrakeSystemControlUnit/1  "FrontLeftWheelBrakePress[Pa]"
  FrontRightWheelBrakePress[Pa]___UNIQUE_1/1 -> __TDD__BrakeSystemControlUnit.FrontRightWheelBrakePress[Pa]/1  "FrontRightWheelBrakePress[Pa]"
  __TDD__BrakeSystemControlUnit.FrontRightWheelBrakePress[Pa]/1 -> __TDO__BrakeSystemControlUnit/2  "FrontRightWheelBrakePress[Pa]"
  RearLeftWheelBrakePress[Pa]___UNIQUE_1/1 -> __TDD__BrakeSystemControlUnit.RearLeftWheelBrakePress[Pa]/1  "RearLeftWheelBrakePress[Pa]"
  __TDD__BrakeSystemControlUnit.RearLeftWheelBrakePress[Pa]/1 -> __TDO__BrakeSystemControlUnit/3  "RearLeftWheelBrakePress[Pa]"
  RearRightWheelBrakePress[Pa]___UNIQUE_1/1 -> __TDD__BrakeSystemControlUnit.RearRightWheelBrakePress[Pa]/1  "RearRightWheelBrakePress[Pa]"
  __TDD__BrakeSystemControlUnit.RearRightWheelBrakePress[Pa]/1 -> __TDO__BrakeSystemControlUnit/4  "RearRightWheelBrakePress[Pa]"
  Rear2LeftWheelBrakePress[Pa]___UNIQUE_1/1 -> __TDD__BrakeSystemControlUnit.Rear2LeftWheelBrakePress[Pa]/1
  __TDD__BrakeSystemControlUnit.Rear2LeftWheelBrakePress[Pa]/1 -> __TDO__BrakeSystemControlUnit/5  "Rear2LeftWheelBrakePress[Pa]"
  Rear2RightWheelBrakePress[Pa]___UNIQUE_1/1 -> __TDD__BrakeSystemControlUnit.Rear2RightWheelBrakePress[Pa]/1
  __TDD__BrakeSystemControlUnit.Rear2RightWheelBrakePress[Pa]/1 -> __TDO__BrakeSystemControlUnit/6  "Rear2RightWheelBrakePress[Pa]"
  Rear3LeftWheelBrakePress[Pa]___UNIQUE_1/1 -> __TDD__BrakeSystemControlUnit.Rear3LeftWheelBrakePress[Pa]/1
  __TDD__BrakeSystemControlUnit.Rear3LeftWheelBrakePress[Pa]/1 -> __TDO__BrakeSystemControlUnit/7  "Rear3LeftWheelBrakePress[Pa]"
  Rear3RightWheelBrakePress[Pa]___UNIQUE_1/1 -> __TDD__BrakeSystemControlUnit.Rear3RightWheelBrakePress[Pa]/1
  __TDD__BrakeSystemControlUnit.Rear3RightWheelBrakePress[Pa]/1 -> __TDO__BrakeSystemControlUnit/8  "Rear3RightWheelBrakePress[Pa]"
  WheelBrakePressActive[0;1]___UNIQUE_1/1 -> __TDD__BrakeSystemControlUnit.WheelBrakePressActive[0;1]/1
  __TDD__BrakeSystemControlUnit.WheelBrakePressActive[0;1]/1 -> __TDO__BrakeSystemControlUnit/9  "WheelBrakePressActive[0;1]"
  YawStabilityControl___UNIQUE_1/1 -> __TDO__BrakeSystemControlUnit.ControlUnit/1  "YawStabilityControl"
  __TDO__BrakeSystemControlUnit.ControlUnit/1 -> __TDO__BrakeSystemControlUnit/10  "ControlUnit"
  AntiLockBrakeSystem___UNIQUE_1/1 -> __TDO__BrakeSystemControlUnit.ControlUnit/2  "AntiLockBrakeSystem"
  __TDO__BrakeSystemControlUnit/1 -> BrakeSystemControlUnit___UNIQUE_1/1  "BrakeSystemControlUnit"

== system PassengerCar/Vehicle/BrakeSystem/BrakeSystemControlUnit/DynaComponentInfo ==

== system PassengerCar/Vehicle/BrakeSystem/BrakeSystemPhysics/BrakeSystemPhysicsOutput ==
  WheelBrakePressActive[0;1]___UNIQUE_1 : Inport  Description=|  PortDimensions=[1]
      | <name>WheelBrakePressActive[0;1]</name>
      | <comment></comment>
  MaxMainBrakePress[Pa]___UNIQUE_1 : Inport  Description=|  Port=2  PortDimensions=[1]
      | <name>MaxMainBrakePress[Pa]</name>
      | <comment></comment>
  MainBrakePress[Pa]___UNIQUE_1 : Inport  Description=|  Port=3  PortDimensions=[1]
      | <name>MainBrakePress[Pa]</name>
      | <comment></comment>
  FrontLeftWheelBrakePress[Pa]___UNIQUE_1 : Inport  Description=|  Port=4  PortDimensions=[1]
      | <name>FrontLeftWheelBrakePress[Pa]</name>
      | <comment></comment>
  FrontRightWheelBrakePress[Pa]___UNIQUE_1 : Inport  Description=|  Port=5  PortDimensions=[1]
      | <name>FrontRightWheelBrakePress[Pa]</name>
      | <comment></comment>
  RearLeftWheelBrakePress[Pa]___UNIQUE_1 : Inport  Description=|  Port=6  PortDimensions=[1]
      | <name>RearLeftWheelBrakePress[Pa]</name>
      | <comment></comment>
  RearRightWheelBrakePress[Pa]___UNIQUE_1 : Inport  Description=|  Port=7  PortDimensions=[1]
      | <name>RearRightWheelBrakePress[Pa]</name>
      | <comment></comment>
  Rear2LeftWheelBrakePress[Pa]___UNIQUE_1 : Inport  Description=|  Port=8  PortDimensions=[1]
      | <name>Rear2LeftWheelBrakePress[Pa]</name>
      | <comment></comment>
  Rear2RightWheelBrakePress[Pa]___UNIQUE_1 : Inport  Description=|  Port=9  PortDimensions=[1]
      | <name>Rear2RightWheelBrakePress[Pa]</name>
      | <comment></comment>
  Rear3LeftWheelBrakePress[Pa]___UNIQUE_1 : Inport  Description=|  Port=10  PortDimensions=[1]
      | <name>Rear3LeftWheelBrakePress[Pa]</name>
      | <comment></comment>
  Rear3RightWheelBrakePress[Pa]___UNIQUE_1 : Inport  Description=|  Port=11  PortDimensions=[1]
      | <name>Rear3RightWheelBrakePress[Pa]</name>
      | <comment></comment>
  __TDD__BrakeSystemPhysics.FrontLeftWheelBrakePress[Pa] : Demux  Outputs=[1]
  __TDD__BrakeSystemPhysics.FrontRightWheelBrakePress[Pa] : Demux  Outputs=[1]
  __TDD__BrakeSystemPhysics.MainBrakePress[Pa] : Demux  Outputs=[1]
  __TDD__BrakeSystemPhysics.MaxMainBrakePress[Pa] : Demux  Outputs=[1]
  __TDD__BrakeSystemPhysics.Rear2LeftWheelBrakePress[Pa] : Demux  Outputs=[1]
  __TDD__BrakeSystemPhysics.Rear2RightWheelBrakePress[Pa] : Demux  Outputs=[1]
  __TDD__BrakeSystemPhysics.Rear3LeftWheelBrakePress[Pa] : Demux  Outputs=[1]
  __TDD__BrakeSystemPhysics.Rear3RightWheelBrakePress[Pa] : Demux  Outputs=[1]
  __TDD__BrakeSystemPhysics.RearLeftWheelBrakePress[Pa] : Demux  Outputs=[1]
  __TDD__BrakeSystemPhysics.RearRightWheelBrakePress[Pa] : Demux  Outputs=[1]
  __TDD__BrakeSystemPhysics.WheelBrakePressActive[0;1] : Demux  Outputs=[1]
  __TDO__BrakeSystemPhysics : BusCreator  Inputs=11
  BrakeSystemPhysics___UNIQUE_1 : Outport  Description=|  PortDimensions=[11]  VectorParamsAs1DForOutWhenUnconnected=off
      | <name>WheelBrakePressActive[0;1]</name>
      | <comment></comment>
  wires:
  WheelBrakePressActive[0;1]___UNIQUE_1/1 -> __TDD__BrakeSystemPhysics.WheelBrakePressActive[0;1]/1  "Active"
  __TDD__BrakeSystemPhysics.WheelBrakePressActive[0;1]/1 -> __TDO__BrakeSystemPhysics/1  "WheelBrakePressActive[0;1]"
  MaxMainBrakePress[Pa]___UNIQUE_1/1 -> __TDD__BrakeSystemPhysics.MaxMainBrakePress[Pa]/1  "MaxMainBrakePress[Pa]"
  __TDD__BrakeSystemPhysics.MaxMainBrakePress[Pa]/1 -> __TDO__BrakeSystemPhysics/2  "MaxMainBrakePress[Pa]"
  MainBrakePress[Pa]___UNIQUE_1/1 -> __TDD__BrakeSystemPhysics.MainBrakePress[Pa]/1  "MainBrakePress[Pa]"
  __TDD__BrakeSystemPhysics.MainBrakePress[Pa]/1 -> __TDO__BrakeSystemPhysics/3  "MainBrakePress[Pa]"
  FrontLeftWheelBrakePress[Pa]___UNIQUE_1/1 -> __TDD__BrakeSystemPhysics.FrontLeftWheelBrakePress[Pa]/1  "FrontLeftWheelBrakePress[Pa]"
  __TDD__BrakeSystemPhysics.FrontLeftWheelBrakePress[Pa]/1 -> __TDO__BrakeSystemPhysics/4  "FrontLeftWheelBrakePress[Pa]"
  FrontRightWheelBrakePress[Pa]___UNIQUE_1/1 -> __TDD__BrakeSystemPhysics.FrontRightWheelBrakePress[Pa]/1  "FrontRightWheelBrakePress[Pa]"
  __TDD__BrakeSystemPhysics.FrontRightWheelBrakePress[Pa]/1 -> __TDO__BrakeSystemPhysics/5  "FrontRightWheelBrakePress[Pa]"
  RearLeftWheelBrakePress[Pa]___UNIQUE_1/1 -> __TDD__BrakeSystemPhysics.RearLeftWheelBrakePress[Pa]/1  "RearLeftWheelBrakePress[Pa]"
  __TDD__BrakeSystemPhysics.RearLeftWheelBrakePress[Pa]/1 -> __TDO__BrakeSystemPhysics/6  "RearLeftWheelBrakePress[Pa]"
  RearRightWheelBrakePress[Pa]___UNIQUE_1/1 -> __TDD__BrakeSystemPhysics.RearRightWheelBrakePress[Pa]/1  "RearRightWheelBrakePress[Pa]"
  __TDD__BrakeSystemPhysics.RearRightWheelBrakePress[Pa]/1 -> __TDO__BrakeSystemPhysics/7  "RearRightWheelBrakePress[Pa]"
  Rear2LeftWheelBrakePress[Pa]___UNIQUE_1/1 -> __TDD__BrakeSystemPhysics.Rear2LeftWheelBrakePress[Pa]/1  "Rear2LeftWheelBrakePress[Pa]"
  __TDD__BrakeSystemPhysics.Rear2LeftWheelBrakePress[Pa]/1 -> __TDO__BrakeSystemPhysics/8  "Rear2LeftWheelBrakePress[Pa]"
  Rear2RightWheelBrakePress[Pa]___UNIQUE_1/1 -> __TDD__BrakeSystemPhysics.Rear2RightWheelBrakePress[Pa]/1  "Rear2RightWheelBrakePress[Pa]"
  __TDD__BrakeSystemPhysics.Rear2RightWheelBrakePress[Pa]/1 -> __TDO__BrakeSystemPhysics/9  "Rear2RightWheelBrakePress[Pa]"
  Rear3LeftWheelBrakePress[Pa]___UNIQUE_1/1 -> __TDD__BrakeSystemPhysics.Rear3LeftWheelBrakePress[Pa]/1  "Rear3LeftWheelBrakePress[Pa]"
  __TDD__BrakeSystemPhysics.Rear3LeftWheelBrakePress[Pa]/1 -> __TDO__BrakeSystemPhysics/10  "Rear3LeftWheelBrakePress[Pa]"
  Rear3RightWheelBrakePress[Pa]___UNIQUE_1/1 -> __TDD__BrakeSystemPhysics.Rear3RightWheelBrakePress[Pa]/1  "Rear3RightWheelBrakePress[Pa]"
  __TDD__BrakeSystemPhysics.Rear3RightWheelBrakePress[Pa]/1 -> __TDO__BrakeSystemPhysics/11  "Rear3RightWheelBrakePress[Pa]"
  __TDO__BrakeSystemPhysics/1 -> BrakeSystemPhysics___UNIQUE_1/1  "BrakeSystemPhysics"

== system PassengerCar/Vehicle/BrakeSystem/BrakeSystemPhysics/DynaComponentInfo ==

== system PassengerCar/Vehicle/BrakeSystem/BrakeSystemPhysics/InputFromBrakeControlCoordinator ==
  fromBrakeControlCoordinator : Inport
  TDBusSelector : BusSelector  OutputSignals=BrakeSwitch[1;3],MainBrakePress[Pa]
  __TDD__BrakeSwitch[1;3] : Demux  Outputs=1
  __TDD__MainBrakePress[Pa] : Demux  Outputs=1
  BrakeSwitch[1;3]___UNIQUE_1 : Outport  Description=|  VectorParamsAs1DForOutWhenUnconnected=off
      | <name>BrakeSwitch[1;3]</name>
      | <comment></comment>
  MainBrakePress[Pa]___UNIQUE_1 : Outport  Description=|  Port=2  VectorParamsAs1DForOutWhenUnconnected=off
      | <name>MainBrakePress[Pa]</name>
      | <comment></comment>
  wires:
  fromBrakeControlCoordinator/1 -> TDBusSelector/1
  TDBusSelector/1 -> __TDD__BrakeSwitch[1;3]/1  "<BrakeSwitch[1;3]>"
  TDBusSelector/2 -> __TDD__MainBrakePress[Pa]/1  "<MainBrakePress[Pa]>"
  __TDD__BrakeSwitch[1;3]/1 -> BrakeSwitch[1;3]___UNIQUE_1/1  "BrakeSwitch[1;3]"
  __TDD__MainBrakePress[Pa]/1 -> MainBrakePress[Pa]___UNIQUE_1/1  "MainBrakePress[Pa]"

== system PassengerCar/Vehicle/BrakeSystem/BrakeSystemPhysics/InputFromCTRL ==
  fromCTRL : Inport
  TDBusSelector : BusSelector  OutputSignals=CTRL.LongitudinalControl.BrakePedalPos[0_1]
  __TDD__BrakePedalPos[0_1] : Demux  Outputs=[1]
  BrakePedalPos[0_1]___UNIQUE_1 : Outport  Description=|  PortDimensions=[1]  VectorParamsAs1DForOutWhenUnconnected=off
      | <name>CTRL.LongitudinalControl.BrakePedalPos[0_1]</name>
      | <comment></comment>
  wires:
  fromCTRL/1 -> TDBusSelector/1
  TDBusSelector/1 -> __TDD__BrakePedalPos[0_1]/1  "<BrakePedalPos[0_1]>"
  __TDD__BrakePedalPos[0_1]/1 -> BrakePedalPos[0_1]___UNIQUE_1/1  "BrakePedalPos[0_1]"

== system PassengerCar/Vehicle/Drivetrain/DrivetrainControlUnit/DrivetrainControlUnitOutput ==
  Gear[-4;20]___UNIQUE_1 : Inport  Description=|  PortDimensions=[1]
      | <name>TransmissionControlUnit.Gear[-4;20]</name>
      | <comment>Gear</comment>
  LockUpClutchPos[0_1]___UNIQUE_1 : Inport  Description=|  Port=2  PortDimensions=[1]
      | <name>TransmissionControlUnit.LockUpClutchPos[0_1]</name>
      | <comment>Lock-up clutch position</comment>
  AutomatedManualClutchPos[0_1]___UNIQUE_1 : Inport  Description=|  Port=3  PortDimensions=[1]
      | <name>TransmissionControlUnit.AutomatedManualClutchPos[0_1]</name>
      | <comment>Clutch position for manual shifting</comment>
  GearTarget[-4;20]___UNIQUE_1 : Inport  Description=|  Port=4  PortDimensions=[1]
      | <name>TransmissionControlUnit.GearTarget[-4;20]</name>
      | <comment>Target gear</comment>
  ASRRequestSwitch[0;2]___UNIQUE_1 : Inport  Description=|  Port=5  PortDimensions=[1]
      | <name>TransmissionControlUnit.ASRRequestSwitch[0;2]</name>
      | <comment></comment>
  ASRTrq[Nm]___UNIQUE_1 : Inport  Description=|  Port=6  PortDimensions=[1]
      | <name>TransmissionControlUnit.ASRTrq[Nm]</name>
      | <comment></comment>
  __SRC__DrivetrainControlUnit.TransmissionControlUnit.MSRRequestSwitch[0;2] : Constant  Value=0.0  OutDataTypeStr=Inherit: Inherit via back propagation
  __SRC__DrivetrainControlUnit.TransmissionControlUnit.MSRTrq[Nm] : Constant  Value=0.0  OutDataTypeStr=Inherit: Inherit via back propagation
  __TDD__DrivetrainControlUnit.TransmissionControlUnit.ASRRequestSwitch[0;2] : Demux  Outputs=[1]
  __TDD__DrivetrainControlUnit.TransmissionControlUnit.ASRTrq[Nm] : Demux  Outputs=[1]
  __TDD__DrivetrainControlUnit.TransmissionControlUnit.AutomatedManualClutchPos[0_1] : Demux  Outputs=[1]
  __TDD__DrivetrainControlUnit.TransmissionControlUnit.GearTarget[-4;20] : Demux  Outputs=[1]
  __TDD__DrivetrainControlUnit.TransmissionControlUnit.Gear[-4;20] : Demux  Outputs=[1]
  __TDD__DrivetrainControlUnit.TransmissionControlUnit.LockUpClutchPos[0_1] : Demux  Outputs=[1]
  __TDO__DrivetrainControlUnit : BusCreator  Inputs=1
  __TDO__DrivetrainControlUnit.TransmissionControlUnit : BusCreator  Inputs=8
  DrivetrainControlUnit___UNIQUE_1 : Outport  Description=|  PortDimensions=[8]  VectorParamsAs1DForOutWhenUnconnected=off
      | <name>TransmissionControlUnit.Gear[-4;20]</name>
      | <comment>Gear</comment>
  wires:
  __TDO__DrivetrainControlUnit/1 -> DrivetrainControlUnit___UNIQUE_1/1  "DrivetrainControlUnit"
  __SRC__DrivetrainControlUnit.TransmissionControlUnit.MSRTrq[Nm]/1 -> __TDO__DrivetrainControlUnit.TransmissionControlUnit/8  "MSRTrq[Nm]"
  __SRC__DrivetrainControlUnit.TransmissionControlUnit.MSRRequestSwitch[0;2]/1 -> __TDO__DrivetrainControlUnit.TransmissionControlUnit/7  "MSRRequestSwitch[0;2]"
  __TDD__DrivetrainControlUnit.TransmissionControlUnit.ASRTrq[Nm]/1 -> __TDO__DrivetrainControlUnit.TransmissionControlUnit/6  "ASRTrq[Nm]"
  ASRTrq[Nm]___UNIQUE_1/1 -> __TDD__DrivetrainControlUnit.TransmissionControlUnit.ASRTrq[Nm]/1
  __TDD__DrivetrainControlUnit.TransmissionControlUnit.ASRRequestSwitch[0;2]/1 -> __TDO__DrivetrainControlUnit.TransmissionControlUnit/5  "ASRRequestSwitch[0;2]"
  ASRRequestSwitch[0;2]___UNIQUE_1/1 -> __TDD__DrivetrainControlUnit.TransmissionControlUnit.ASRRequestSwitch[0;2]/1
  __TDD__DrivetrainControlUnit.TransmissionControlUnit.GearTarget[-4;20]/1 -> __TDO__DrivetrainControlUnit.TransmissionControlUnit/4  "GearTarget[-4;20]"
  GearTarget[-4;20]___UNIQUE_1/1 -> __TDD__DrivetrainControlUnit.TransmissionControlUnit.GearTarget[-4;20]/1
  __TDD__DrivetrainControlUnit.TransmissionControlUnit.AutomatedManualClutchPos[0_1]/1 -> __TDO__DrivetrainControlUnit.TransmissionControlUnit/3  "AutomatedManualClutchPos[0_1]"
  AutomatedManualClutchPos[0_1]___UNIQUE_1/1 -> __TDD__DrivetrainControlUnit.TransmissionControlUnit.AutomatedManualClutchPos[0_1]/1
  __TDD__DrivetrainControlUnit.TransmissionControlUnit.LockUpClutchPos[0_1]/1 -> __TDO__DrivetrainControlUnit.TransmissionControlUnit/2  "LockUpClutchPos[0_1]"
  LockUpClutchPos[0_1]___UNIQUE_1/1 -> __TDD__DrivetrainControlUnit.TransmissionControlUnit.LockUpClutchPos[0_1]/1
  __TDO__DrivetrainControlUnit.TransmissionControlUnit/1 -> __TDO__DrivetrainControlUnit/1  "TransmissionControlUnit"
  __TDD__DrivetrainControlUnit.TransmissionControlUnit.Gear[-4;20]/1 -> __TDO__DrivetrainControlUnit.TransmissionControlUnit/1  "Gear[-4;20]"
  Gear[-4;20]___UNIQUE_1/1 -> __TDD__DrivetrainControlUnit.TransmissionControlUnit.Gear[-4;20]/1

== system PassengerCar/Vehicle/Drivetrain/DrivetrainControlUnit/DynaComponentInfo ==

== system PassengerCar/Vehicle/Drivetrain/DrivetrainControlUnit/InputFromCTRL ==
  fromCTRL : Inport
  TDBusSelector : BusSelector  OutputSignals=CTRL.LongitudinalControl.TransmissionLoad[0_1],CTRL.LongitudinalControl.IntendedEngTrqActive[0;1],CTRL.LongitudinalControl.AccPedalPos[0_1],CTRL.LongitudinalControl.InitialGear[-4;20],CTRL.LongitudinalControl.MaxGear[-4;20],CTRL.LongitudinalControl.MinGear[-4;20],CTRL.LongitudinalControl.ShiftingProgramSelection[-],CTRL.LongitudinalControl.KickdownSwitch[0;1]
  __TDD__AccPedalPos[0_1] : Demux  Outputs=[1]
  __TDD__InitialGear[-4;20] : Demux  Outputs=[1]
  __TDD__IntendedEngTrqActive[0;1] : Demux  Outputs=[1]
  __TDD__KickdownSwitch[0;1] : Demux  Outputs=[1]
  __TDD__MaxGear[-4;20] : Demux  Outputs=[1]
  __TDD__MinGear[-4;20] : Demux  Outputs=[1]
  __TDD__ShiftingProgramSelection[-] : Demux  Outputs=[1]
  __TDD__TransmissionLoad[0_1] : Demux  Outputs=[1]
  TransmissionLoad[0_1]___UNIQUE_1 : Outport  Description=|  PortDimensions=[1]  VectorParamsAs1DForOutWhenUnconnected=off
      | <name>CTRL.LongitudinalControl.TransmissionLoad[0_1]</name>
      | <comment></comment>
  IntendedEngTrqActive[0;1]___UNIQUE_1 : Outport  Description=|  Port=2  PortDimensions=[1]  VectorParamsAs1DForOutWhenUnconnected=off
      | <name>CTRL.LongitudinalControl.IntendedEngTrqActive[0;1]</name>
      | <comment></comment>
  AccPedalPos[0_1]___UNIQUE_1 : Outport  Description=|  Port=3  PortDimensions=[1]  VectorParamsAs1DForOutWhenUnconnected=off
      | <name>CTRL.LongitudinalControl.AccPedalPos[0_1]</name>
      | <comment></comment>
  InitialGear[-4;20]___UNIQUE_1 : Outport  Description=|  Port=4  PortDimensions=[1]  VectorParamsAs1DForOutWhenUnconnected=off
      | <name>CTRL.LongitudinalControl.InitialGear[-4;20]</name>
      | <comment></comment>
  MaxGear[-4;20]___UNIQUE_1 : Outport  Description=|  Port=5  PortDimensions=[1]  VectorParamsAs1DForOutWhenUnconnected=off
      | <name>CTRL.LongitudinalControl.MaxGear[-4;20]</name>
      | <comment>Maximum gear</comment>
  MinGear[-4;20]___UNIQUE_1 : Outport  Description=|  Port=6  PortDimensions=[1]  VectorParamsAs1DForOutWhenUnconnected=off
      | <name>CTRL.LongitudinalControl.MinGear[-4;20]</name>
      | <comment>Minimum gear</comment>
  ShiftingProgramSelection[-]___UNIQUE_1 : Outport  Description=|  Port=7  PortDimensions=[1]  VectorParamsAs1DForOutWhenUnconnected=off
      | <name>CTRL.LongitudinalControl.ShiftingProgramSelection[-]</name>
      | <comment>Shifting program selection</comment>
  KickdownSwitch[0;1]___UNIQUE_1 : Outport  Description=|  Port=8  PortDimensions=[1]  VectorParamsAs1DForOutWhenUnconnected=off
      | <name>CTRL.LongitudinalControl.KickdownSwitch[0;1]</name>
      | <comment>Kickdown switch</comment>
  wires:
  __TDD__KickdownSwitch[0;1]/1 -> KickdownSwitch[0;1]___UNIQUE_1/1  "KickdownSwitch[0;1]"
  __TDD__ShiftingProgramSelection[-]/1 -> ShiftingProgramSelection[-]___UNIQUE_1/1  "ShiftingProgramSelection[-]"
  __TDD__MinGear[-4;20]/1 -> MinGear[-4;20]___UNIQUE_1/1  "MinGear[-4;20]"
  __TDD__MaxGear[-4;20]/1 -> MaxGear[-4;20]___UNIQUE_1/1  "MaxGear[-4;20]"
  __TDD__InitialGear[-4;20]/1 -> InitialGear[-4;20]___UNIQUE_1/1  "InitialGear[-4;20]"
  __TDD__AccPedalPos[0_1]/1 -> AccPedalPos[0_1]___UNIQUE_1/1  "AccPedalPos[0_1]"
  __TDD__IntendedEngTrqActive[0;1]/1 -> IntendedEngTrqActive[0;1]___UNIQUE_1/1  "IntendedEngTrqActive[0;1]"
  __TDD__TransmissionLoad[0_1]/1 -> TransmissionLoad[0_1]___UNIQUE_1/1  "TransmissionLoad[0_1]"
  TDBusSelector/8 -> __TDD__KickdownSwitch[0;1]/1  "<KickdownSwitch[0;1]>"
  TDBusSelector/7 -> __TDD__ShiftingProgramSelection[-]/1  "<ShiftingProgramSelection[-]>"
  TDBusSelector/6 -> __TDD__MinGear[-4;20]/1  "<MinGear[-4;20]>"
  TDBusSelector/5 -> __TDD__MaxGear[-4;20]/1  "<MaxGear[-4;20]>"
  TDBusSelector/4 -> __TDD__InitialGear[-4;20]/1  "<InitialGear[-4;20]>"
  TDBusSelector/3 -> __TDD__AccPedalPos[0_1]/1  "<AccPedalPos[0_1]>"
  TDBusSelector/2 -> __TDD__IntendedEngTrqActive[0;1]/1  "<IntendedEngTrqActive[0;1]>"
  TDBusSelector/1 -> __TDD__TransmissionLoad[0_1]/1  "<TransmissionLoad[0_1]>"
  fromCTRL/1 -> TDBusSelector/1
